simulink model "plant_control_1"  (R2023a)
settings: Solver=FixedStepAuto  StartTime=0.0  StopTime=10.0  FixedStep=0.01  RelTol=1e-3
values from neighbouring files (symbols this model uses):
  g = 9.81    [control_law_design.m]
  Kp_p = 7.1614    [control_law_design.m]
  Kp_q = 7.1614    [control_law_design.m]
  Kp_r = 3.3884    [control_law_design.m]
  m = 10    [control_law_design.m]
  omega_ref = [1, 1, 1]    [control_law_design.m]
  s = tf('s')    [control_law_design.m]    (also in untitled.m)
libraries: slctrlblks x6, simulink_extras x4, shared6dof x1
settings Model: Creator=timme  LastModifiedBy=timme
settings OptimizationCC: BlockReduction=off  DefaultParameterBehavior=Inlined  BufferReuse=off

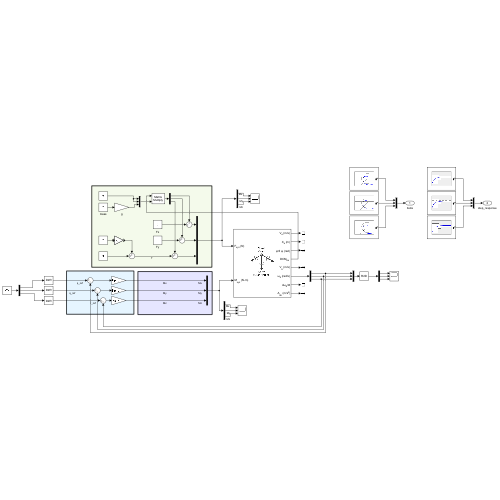
[thumbnail: Simulink's stored preview of the top-level diagram]
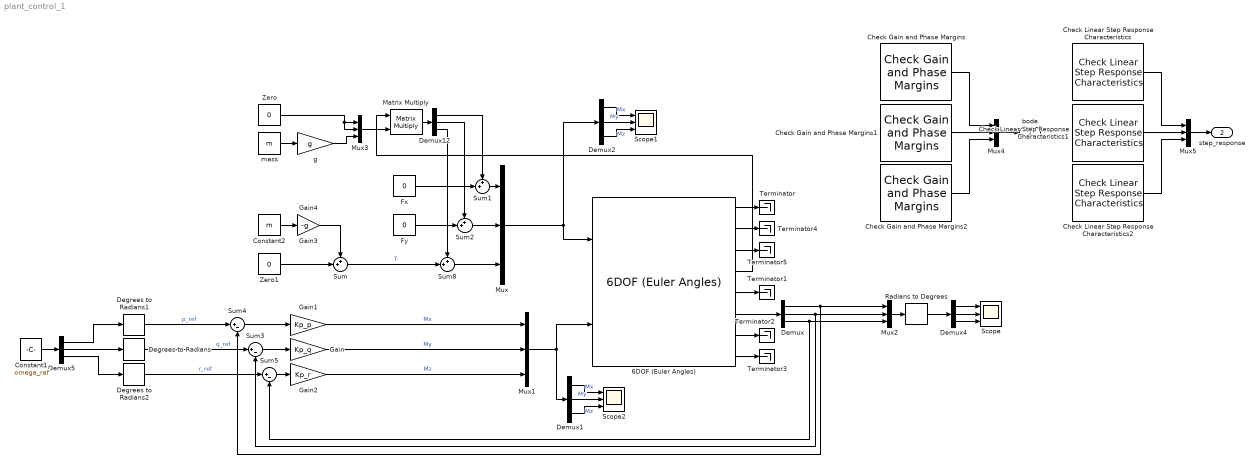
== system plant_control_1 ==
  6DOF (Euler Angles) : shared6dof/6DOF (Euler Angles)  units=Metric (MKS)  mtype=Fixed  rep=Euler Angles  xme_0=[0 0 0]  Vm_0=[0 0 0]  eul_0=[0 0 0]  pm_0=[0 0 0]  mass_0=m  mass_e=0.5  mass_f=2.0  inertia=I  inertia_e=eye(3)  inertia_f=2*eye(3)  k_quat=1.0  vre_flag=on  abi_flag=off  aMode=0  xme_statename=''  Vm_statename=''  eul_statename=''  quat_statename=''  pm_statename=''  mass_statename=''
  Check Gain and Phase Margins : slctrlblks/Model Verification/Check Gain and Phase Margins  InstantiateOnLoad=on  SaveOperatingPoints=off  LinearizationIOs={'/Demux', 1, 'out', 'on', '';'/Degrees to Radians1', 1, 'in', 'on', ''}  LinearizeAt=SnapshotTimes  SnapshotTimes=[0]  TriggerType=rising  SampleTime=auto  RateConversionMethod=zoh  PreWarpFreq=10  UseExactDelayModel=off  UseFullBlockNameLabels=off  UseBusSignalLabels=off  enabled=on  stopWhenAssertionFail=off  export=on  ViewDlgPos=[100 200 510 390]  LaunchViewOnOpen=off  OpenViewOnLoad=off  FrequencyUnits=rad/s  MagnitudeUnits=dB  PhaseUnits=deg  TimeUnits=seconds  EnableMargins=on  GainMargin=200  PhaseMargin=90  PlotType=table  FeedbackSign=-1
      settings: SaveToWorkspace=on  SaveName=sys1_1_1
  Check Gain and Phase Margins1 : slctrlblks/Model Verification/Check Gain and Phase Margins  InstantiateOnLoad=on  SaveOperatingPoints=off  LinearizationIOs={'/Degrees to Radians', 1, 'in', 'on', '';'/Demux', 2, 'out', 'on', ''}  LinearizeAt=SnapshotTimes  SnapshotTimes=[0]  TriggerType=rising  SampleTime=auto  RateConversionMethod=zoh  PreWarpFreq=10  UseExactDelayModel=off  UseFullBlockNameLabels=off  UseBusSignalLabels=off  enabled=on  stopWhenAssertionFail=off  export=on  ViewDlgPos=[100 200 510 390]  LaunchViewOnOpen=off  OpenViewOnLoad=off  FrequencyUnits=rad/s  MagnitudeUnits=dB  PhaseUnits=deg  TimeUnits=seconds  EnableMargins=on  GainMargin=200  PhaseMargin=90  PlotType=table  FeedbackSign=-1
      settings: SaveToWorkspace=on  SaveName=sys1_2_1
  Check Gain and Phase Margins2 : slctrlblks/Model Verification/Check Gain and Phase Margins  InstantiateOnLoad=on  SaveOperatingPoints=off  LinearizationIOs={'/Demux', 3, 'out', 'on', '';'/Degrees to Radians2', 1, 'in', 'on', ''}  LinearizeAt=SnapshotTimes  SnapshotTimes=[0]  TriggerType=rising  SampleTime=auto  RateConversionMethod=zoh  PreWarpFreq=10  UseExactDelayModel=off  UseFullBlockNameLabels=off  UseBusSignalLabels=off  enabled=on  stopWhenAssertionFail=off  export=on  ViewDlgPos=[100 200 510 390]  LaunchViewOnOpen=off  OpenViewOnLoad=off  FrequencyUnits=rad/s  MagnitudeUnits=dB  PhaseUnits=deg  TimeUnits=seconds  EnableMargins=on  GainMargin=200  PhaseMargin=90  PlotType=table  FeedbackSign=-1
      settings: SaveToWorkspace=on  SaveName=sys1_3_1
  Check Linear Step Response Characteristics : slctrlblks/Model Verification/Check Linear Step Response Characteristics  InstantiateOnLoad=on  SaveOperatingPoints=off  LinearizationIOs={'/Demux5', 1, 'in', 'on', '';'/Demux4', 1, 'out', 'on', ''}  LinearizeAt=SnapshotTimes  SnapshotTimes=[0]  TriggerType=rising  SampleTime=auto  RateConversionMethod=zoh  PreWarpFreq=10  UseExactDelayModel=off  UseFullBlockNameLabels=off  UseBusSignalLabels=off  enabled=on  stopWhenAssertionFail=off  export=on  ViewDlgPos=[1 49 1536 740.8]  OpenViewOnLoad=off  LaunchViewOnOpen=off  FrequencyUnits=rad/s  MagnitudeUnits=dB  PhaseUnits=deg  TimeUnits=seconds  EnableStepResponseBound=on  FinalValue=1  RiseTime=1  PercentRise=80  SettlingTime=7  PercentSettling=1  PercentOvershoot=1  PercentUndershoot=1
      settings: SaveToWorkspace=on  SaveName=sys1_1_2
  Check Linear Step Response Characteristics1 : slctrlblks/Model Verification/Check Linear Step Response Characteristics  InstantiateOnLoad=on  SaveOperatingPoints=off  LinearizationIOs={'/Demux5', 2, 'in', 'on', '';'/Demux4', 2, 'out', 'on', ''}  LinearizeAt=SnapshotTimes  SnapshotTimes=[0]  TriggerType=rising  SampleTime=auto  RateConversionMethod=zoh  PreWarpFreq=10  UseExactDelayModel=off  UseFullBlockNameLabels=off  UseBusSignalLabels=off  enabled=on  stopWhenAssertionFail=off  export=on  ViewDlgPos=[1 49 1536 740.8]  OpenViewOnLoad=off  LaunchViewOnOpen=off  FrequencyUnits=rad/s  MagnitudeUnits=dB  PhaseUnits=deg  TimeUnits=seconds  EnableStepResponseBound=on  FinalValue=1  RiseTime=1  PercentRise=80  SettlingTime=7  PercentSettling=1  PercentOvershoot=1  PercentUndershoot=1
      settings: SaveToWorkspace=on  SaveName=sys1_2_2
  Check Linear Step Response Characteristics2 : slctrlblks/Model Verification/Check Linear Step Response Characteristics  InstantiateOnLoad=on  SaveOperatingPoints=off  LinearizationIOs={'/Demux5', 3, 'in', 'on', '';'/Demux4', 3, 'out', 'on', ''}  LinearizeAt=SnapshotTimes  SnapshotTimes=[0]  TriggerType=rising  SampleTime=auto  RateConversionMethod=zoh  PreWarpFreq=10  UseExactDelayModel=off  UseFullBlockNameLabels=off  UseBusSignalLabels=off  enabled=on  stopWhenAssertionFail=off  export=on  ViewDlgPos=[1 49 1536 740.8]  OpenViewOnLoad=off  LaunchViewOnOpen=off  FrequencyUnits=rad/s  MagnitudeUnits=dB  PhaseUnits=deg  TimeUnits=seconds  EnableStepResponseBound=on  FinalValue=1  RiseTime=1  PercentRise=80  SettlingTime=7  PercentSettling=1  PercentOvershoot=1  PercentUndershoot=1
      settings: SaveToWorkspace=on  SaveName=sys1_3_2
  Constant1 : Constant  Value=omega_ref
  Constant2 : Constant  Value=m
  Degrees to Radians : simulink_extras/Transformations/Degrees to Radians
  Degrees to Radians1 : simulink_extras/Transformations/Degrees to Radians
  Degrees to Radians2 : simulink_extras/Transformations/Degrees to Radians
  Demux{,1..2,4..5,12} (6 alike) : Demux  Outputs=3
  Fx : Constant  Value=0
  Fy : Constant  Value=0
  Gain : Gain  Gain=Kp_q
  Gain1 : Gain  Gain=Kp_p
  Gain2 : Gain  Gain=Kp_r
  Gain3 : Gain  Gain=-g
  Gain4 : Gain  Gain=-g
  Matrix Multiply : Product  Inputs=**  Multiplication=Matrix(*)
  Mux{,1..5} (6 alike) : Mux  Inputs=3
  Radians to Degrees : simulink_extras/Transformations/Radians to Degrees
  Scope : Scope  NumInputPorts=3
  Scope1 : Scope  NumInputPorts=3
  Scope2 : Scope  NumInputPorts=3
  Sum{,1..2,8} (4 alike) : Sum  Inputs=++|
  Sum3 : Sum  Inputs=|+-
  Sum4 : Sum  Inputs=|+-
  Sum5 : Sum  Inputs=|+-
  Terminator{,1..5} (6 alike) : Terminator
  Zero : Constant  Value=0  OutDataTypeStr=Inherit: Inherit via back propagation
  Zero1 : Constant  Value=0  OutDataTypeStr=Inherit: Inherit via back propagation
  g : Gain  Gain=g
  mass : Constant  Value=m
  bode : Outport
  step_response : Outport  Port=2
  wires:
  Mux1/1 -> 6DOF (Euler Angles)/2, Demux1/1
  6DOF (Euler Angles)/5 -> Terminator1/1
  6DOF (Euler Angles)/7 -> Terminator2/1
  6DOF (Euler Angles)/8 -> Terminator3/1
  Demux1/2 -> Scope2/2  "My"
  Demux1/1 -> Scope2/1  "Mx"
  Demux1/3 -> Scope2/3  "Mz"
  Zero1/1 -> Sum/2
  mass/1 -> g/1
  Zero/1 -> Mux3/1, Mux3/2
  Sum2/1 -> Mux/2
  6DOF (Euler Angles)/4 -> Matrix Multiply/1
  Fx/1 -> Sum1/2
  Demux12/1 -> Sum1/1
  g/1 -> Mux3/3
  Gain3/1 -> Sum/1
  Sum8/1 -> Mux/3
  Matrix Multiply/1 -> Demux12/1
  Sum/1 -> Sum8/2  "T"
  Sum1/1 -> Mux/1
  Demux12/3 -> Sum8/1
  Fy/1 -> Sum2/2
  Mux3/1 -> Matrix Multiply/2
  Demux12/2 -> Sum2/1
  Mux/1 -> Demux2/1, 6DOF (Euler Angles)/1
  Demux2/1 -> Scope1/1  "Mx"
  Demux2/2 -> Scope1/2  "My"
  Demux2/3 -> Scope1/3  "Mz"
  6DOF (Euler Angles)/6 -> Demux/1
  6DOF (Euler Angles)/3 -> Terminator5/1
  6DOF (Euler Angles)/1 -> Terminator/1
  6DOF (Euler Angles)/2 -> Terminator4/1
  Gain2/1 -> Mux1/3  "Mz"
  Sum5/1 -> Gain2/1
  Demux/1 -> Mux2/1, Sum4/2
  Sum4/1 -> Gain1/1
  Degrees to Radians/1 -> Sum3/1  "q_ref"
  Gain/1 -> Mux1/2  "My"
  Demux/3 -> Sum5/2, Mux2/3
  Degrees to Radians2/1 -> Sum5/1  "r_ref"
  Degrees to Radians1/1 -> Sum4/1  "p_ref"
  Sum3/1 -> Gain/1
  Gain1/1 -> Mux1/1  "Mx"
  Demux/2 -> Mux2/2, Sum3/2
  Demux5/2 -> Degrees to Radians/1
  Mux2/1 -> Radians to Degrees/1
  Radians to Degrees/1 -> Demux4/1
  Demux4/2 -> Scope/2
  Demux4/1 -> Scope/1
  Demux4/3 -> Scope/3
  Check Gain and Phase Margins/1 -> Mux4/1
  Check Gain and Phase Margins1/1 -> Mux4/2
  Check Gain and Phase Margins2/1 -> Mux4/3
  Mux4/1 -> bode/1
  Constant2/1 -> Gain3/1
  Constant1/1 -> Demux5/1
  Demux5/3 -> Degrees to Radians2/1
  Demux5/1 -> Degrees to Radians1/1
  Mux5/1 -> step_response/1
  Check Linear Step Response Characteristics1/1 -> Mux5/2
  Check Linear Step Response Characteristics2/1 -> Mux5/3
  Check Linear Step Response Characteristics/1 -> Mux5/1
